simulink model "OLD_dec_fir_snb"  (R2012b)
settings: Solver=FixedStepDiscrete  SolverMode=SingleTasking  StartTime=0.0  StopTime=10000  FixedStep=1  RelTol=1e-3
libraries: xbsIndex_r4 x1157, casper_library_misc x5, xps_library x1
(part 1 of 9)
settings Model: Creator=paulp  LastModifiedBy=paulp
settings DataIOCC: LimitDataPoints=off
settings OptimizationCC: SimCompilerOptimization=On

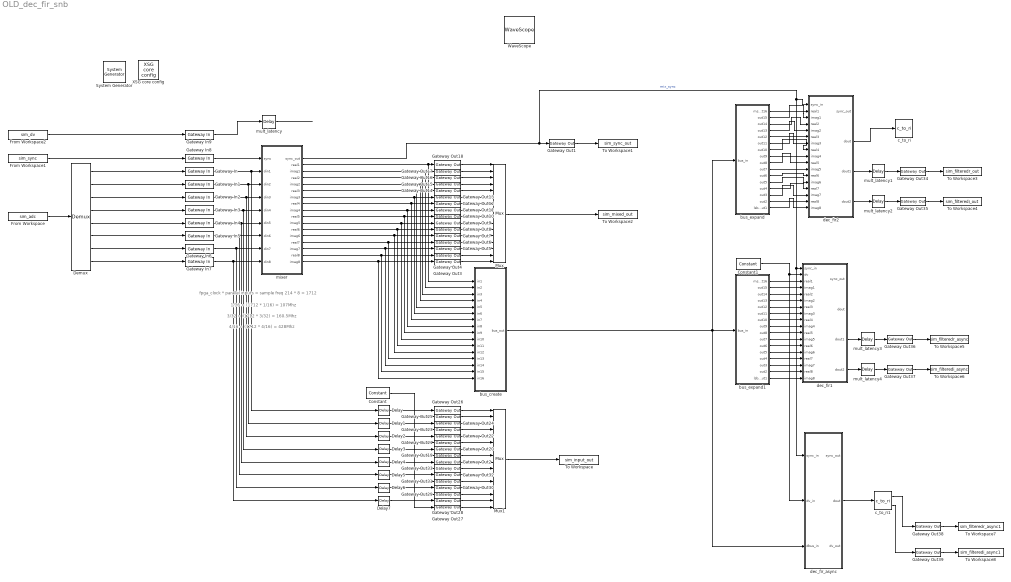
== system OLD_dec_fir_snb ==
  note: fpga_clock * parallel inputs = sample freq
      | 214 * 8 = 1712
  note: 1/16 = (1712 * 1/16) = 107Mhz
  note: 3/32 = (1712 * 3/32) = 160.5Mhz
  note: 4/16 = (1712 * 4/16) = 428Mhz
  " System Generator" : xbsIndex_r4/ System Generator  Tag=genX  xilinxfamily=virtex6  part=xc6vsx475t  speed=-1  package=ff1759  synthesis_tool=XST  clock_wrapper=Clock Enables  directory=./netlist  proj_type=Project Navigator  Synth_file=XST Defaults  Impl_file=ISE Defaults  testbench=off  simulink_period=1  sysclk_period=10  dcm_input_clock_period=10  incr_netlist=off  trim_vbits=Everywhere in SubSystem  dbl_ovrd=According to Block Masks  core_generation=According to Block Masks  run_coregen=off  deprecated_control=off  eval_field=0  block_type=sysgen
  Constant : xbsIndex_r4/Constant  const=0  gui_display_data_type=Fixed-point  arith_type=Signed (2's comp)  n_bits=10  bin_pt=9  preci_type=Single  exp_width=8  frac_width=24  explicit_period=on  period=1  equ=P=C  opselect=C  inp2=PCIN>>17  opr=+  inp1=P  carry=CIN  dbl_ovrd=off  block_type=constant
  Constant1 : xbsIndex_r4/Constant  const=1  gui_display_data_type=Boolean  arith_type=Boolean  n_bits=10  bin_pt=9  preci_type=Single  exp_width=8  frac_width=24  explicit_period=on  period=1  equ=P=C  opselect=C  inp2=PCIN>>17  opr=+  inp1=P  carry=CIN  dbl_ovrd=off  block_type=constant
  Delay{,1..7} (8 alike) : xbsIndex_r4/Delay  rst=off  infoeditControl=Selection of Reset will increase slice count due to use of real FFs and instead of SRLs  en=off  latency=1  dbl_ovrd=off  reg_retiming=off  block_type=delay
  Demux : Demux  Outputs=8
  From Workspace : FromWorkspace  VariableName=sim_adc  SampleTime=1  Interpolate=off  OutputAfterFinalValue=Setting to zero
  From Workspace1 : FromWorkspace  VariableName=sim_sync  SampleTime=1  Interpolate=off  OutputAfterFinalValue=Setting to zero
  From Workspace2 : FromWorkspace  VariableName=sim_dv  SampleTime=1  Interpolate=off  OutputAfterFinalValue=Setting to zero
  Gateway In{,1..7} (8 alike) : xbsIndex_r4/Gateway In  gui_display_data_type=Fixed-point  arith_type="Signed  (2's comp)"  n_bits=10  bin_pt=9  preci_type=Single  exp_width=8  frac_width=24  quantization="Round  (unbiased: +/- Inf)"  overflow=Saturate  period=1  dbl_ovrd=off  timing_constraint=None  locs_specified=off  LOCs={}  UseAsADC=off  ADCChannel='1'  inherit_from_input=off  hdl_port=on  block_type=gatewayin
  Gateway In8 : xbsIndex_r4/Gateway In  gui_display_data_type=Boolean  arith_type=Boolean  n_bits=10  bin_pt=9  preci_type=Single  exp_width=8  frac_width=24  quantization="Round  (unbiased: +/- Inf)"  overflow=Saturate  period=1  dbl_ovrd=off  timing_constraint=None  locs_specified=off  LOCs={}  UseAsADC=off  ADCChannel='1'  inherit_from_input=off  hdl_port=on  block_type=gatewayin
  Gateway In9 : xbsIndex_r4/Gateway In  gui_display_data_type=Boolean  arith_type=Boolean  n_bits=10  bin_pt=9  preci_type=Single  exp_width=8  frac_width=24  quantization="Round  (unbiased: +/- Inf)"  overflow=Saturate  period=1  dbl_ovrd=off  timing_constraint=None  locs_specified=off  LOCs={}  UseAsADC=off  ADCChannel='1'  inherit_from_input=off  hdl_port=on  block_type=gatewayin
  Gateway Out{1..39} (39 alike) : xbsIndex_r4/Gateway Out  inherit_from_input=off  hdl_port=off  timing_constraint=None  locs_specified=off  LOCs={}  UseAsDAC=off  DACChannel='1'  block_type=gatewayout
  Mux : Mux  Inputs=16
  Mux1 : Mux  Inputs=16
  To Workspace : ToWorkspace  VariableName=sim_input_out  SampleTime=1  SaveFormat=Structure With Time
  To Workspace1 : ToWorkspace  VariableName=sim_sync_out  SampleTime=1  SaveFormat=Structure With Time
  To Workspace2 : ToWorkspace  VariableName=sim_mixed_out  SampleTime=1  SaveFormat=Structure With Time
  To Workspace3 : ToWorkspace  VariableName=sim_filteredr_out  SampleTime=1  SaveFormat=Structure With Time
  To Workspace4 : ToWorkspace  VariableName=sim_filteredi_out  SampleTime=1  SaveFormat=Structure With Time
  To Workspace5 : ToWorkspace  VariableName=sim_filteredr_async  SampleTime=1  SaveFormat=Structure With Time
  To Workspace6 : ToWorkspace  VariableName=sim_filteredi_async  SampleTime=1  SaveFormat=Structure With Time
  To Workspace7 : ToWorkspace  VariableName=sim_filteredr_async1  SampleTime=1  SaveFormat=Structure With Time
  To Workspace8 : ToWorkspace  VariableName=sim_filteredi_async1  SampleTime=1  SaveFormat=Structure With Time
  WaveScope : xbsIndex_r4/WaveScope  block_type=wavescope
  XSG core config : xps_library/XSG core config  Tag=xps:xsg  hw_sys=ROACH2:sx475t  clk_src=sys_clk  ROACH_clk_src=sys_clk  ROACH2_clk_src=sys_clk  MKDIG_clk_src=sys_clk  clk_rate=214  sample_period=1  synthesis_tool=XST
  bus_create : Subsystem  AncestorBlock=casper_library_flow_control/bus_create  mask(bus_create){inputNum=16}
      mask prompts: inputNum "Number of inputs:"
      mask init:
      | bus_create_init(gcb,...
      |     'inputNum', inputNum);
  bus_expand : Subsystem  AncestorBlock=casper_library_flow_control/bus_expand  mask(bus_expand){mode=divisions of equal size, outputNum=16, outputWidth=20, outputBinaryPt=18, outputArithmeticType=1, show_format=off, outputToWorkspace=off, variablePrefix=out, outputToModelAsWell=on}
      mask prompts: outputNum "Number of outputs:"; outputWidth "Output width:"; outputBinaryPt "Output binary point position:"; outputArithmeticType "Output arithmetic type (ufix=0, fix=1, bool=2):"; show_format "Print format string?"; outputToWorkspace "Output to workspace?"; variablePrefix "Variable name prefix:"; outputToModelAsWell "Output to model as well?"
      mask help:
      | Expands a 'bus' made using a bus_create or Xilinx
      | concat block.
      | The input will be divided into the specified number
      | of outputs with the specified arithmetic types.
      | Divisions are made from most significant bit.
      mask init:
      | bus_expand_init(gcb,...
      |     'mode', mode, ...
      |     'outputNum', outputNum, ...
      |     'outputWidth', outputWidth, ...
      |     'outputBinaryPt', outputBinaryPt, ...
      |     'outputArithmeticType', outputArithmeticType, ...
      |     'show_format', show_format, ...
      |     'outputToWorkspace', outputToWorkspace, ...
      |     'variablePrefix', variablePrefix, ...
      |     'outputToModelAsWell', outputToModelAsWell);
      settings: AttributesFormatString=16 outputs
      mask TypeOptions mode: divisions of equal size | divisions of arbitrary size
      mask Callback mode: bus_expand_callback();
      mask Callback outputWidth: bus_expand_callback();
      mask Callback outputToWorkspace: bus_expand_callback();
  bus_expand1 : Subsystem  AncestorBlock=casper_library_flow_control/bus_expand  mask(bus_expand){mode=divisions of equal size, outputNum=16, outputWidth=20, outputBinaryPt=18, outputArithmeticType=1, show_format=off, outputToWorkspace=off, variablePrefix=out, outputToModelAsWell=on}
      mask prompts: outputNum "Number of outputs:"; outputWidth "Output width:"; outputBinaryPt "Output binary point position:"; outputArithmeticType "Output arithmetic type (ufix=0, fix=1, bool=2):"; show_format "Print format string?"; outputToWorkspace "Output to workspace?"; variablePrefix "Variable name prefix:"; outputToModelAsWell "Output to model as well?"
      mask help:
      | Expands a 'bus' made using a bus_create or Xilinx
      | concat block.
      | The input will be divided into the specified number
      | of outputs with the specified arithmetic types.
      | Divisions are made from most significant bit.
      mask init: same as OLD_dec_fir_snb/bus_expand
      settings: AttributesFormatString=16 outputs
      mask TypeOptions mode: divisions of equal size | divisions of arbitrary size
      mask Callback mode: bus_expand_callback();
      mask Callback outputWidth: bus_expand_callback();
      mask Callback outputToWorkspace: bus_expand_callback();
  c_to_ri : casper_library_misc/c_to_ri  n_bits=32  bin_pt=31
      settings: AttributesFormatString=32_31 r/i
  c_to_ri1 : casper_library_misc/c_to_ri  n_bits=20  bin_pt=19
      settings: AttributesFormatString=20_19 r/i
  dec_fir1 : Subsystem  Tag=casper:dec_fir  mask(dec_fir){n_inputs=8, coeff=|, n_bits=32, quantization=Round  (unbiased: +/- Inf), add_latency=1, mult_latency=2, conv_latency=2, coeff_bit_width=25, coeff_bin_pt=23, absorb_adders=off, adder_imp=Behavioral}
      mask coeff=|
      | [0.00192582027899352	0.00270863257211452	0.00460769136115305	0.00722478458223097	0.0106379289193187	0.0148769089466709	0.0199095287177559	0.0256326100943865	0.0318695836606276	0.0383758422175682	0.0448521125466397	0.0509650671776680	0.0563733906596148	0.0607566857782212	0.0638440864370335	0.0654393260500031	0.0654393260500031	0.0638440864370335	0.0607566857782212	0.0563733906596148	0.0509650671776680	0.0448521125466397	0.0383758422175682	0.0318695836606276	0.0256326100943865	0.0199095287177559	0.0148769089466709	0.0106379289193187	0.00722478458223097	0.00460769136115305	0.00270863257211452	0.00192582027899352
      | ]
      mask prompts: n_inputs "Number of Parallel Streams"; coeff "Coefficients"; n_bits "Bit Width Out"; quantization "Quantization Behavior"; add_latency "Add Latency"; mult_latency "Mult Latency"; conv_latency "Convert latency"; coeff_bit_width "Coefficient bit width"; coeff_bin_pt "Coefficient binary point"; absorb_adders "Absorb adders into DSP slices"; adder_imp "Adder implementation"
      mask help: FIR filter which can handle multiple time samples in parallel and decimates down to 1 time sample. If coefficients are symmetric, will automatically fold before multiplying.
      mask init:
      | % dec_fir_init(gcb, ...
      | %     'n_inputs', n_inputs, ...
      | %     'coeff', coeff, ...
      | %     'n_bits', n_bits, ...
      | %     'quantization', quantization, ...
      | %     'add_latency', add_latency, ...
      | %     'mult_latency', mult_latency, ...
      | %     'conv_latency', conv_latency, ...
      | %     'coeff_bit_width', coeff_bit_width, ...
      | %     'coeff_bin_pt', coeff_bin_pt, ...
      | %     'absorb_adders', absorb_adders, ...
      | %     'adder_imp', adder_imp);
      settings: AttributesFormatString=|
      | 32 taps
      | 32_31 r/i
      mask TypeOptions quantization: Truncate | Round  (unbiased: +/- Inf) | Round  (unbiased: Even Values)
      mask TypeOptions adder_imp: Behavioral | Fabric | DSP48
  dec_fir2 : Subsystem  Tag=casper:dec_fir  AncestorBlock=casper_library_downconverter/dec_fir  mask(dec_fir){n_inputs=8, coeff=|, n_bits=32, quantization=Round  (unbiased: +/- Inf), add_latency=1, mult_latency=2, conv_latency=2, coeff_bit_width=25, coeff_bin_pt=23, absorb_adders=off, adder_imp=Behavioral}
      mask coeff=|
      | [0.00192582027899352	0.00270863257211452	0.00460769136115305	0.00722478458223097	0.0106379289193187	0.0148769089466709	0.0199095287177559	0.0256326100943865	0.0318695836606276	0.0383758422175682	0.0448521125466397	0.0509650671776680	0.0563733906596148	0.0607566857782212	0.0638440864370335	0.0654393260500031	0.0654393260500031	0.0638440864370335	0.0607566857782212	0.0563733906596148	0.0509650671776680	0.0448521125466397	0.0383758422175682	0.0318695836606276	0.0256326100943865	0.0199095287177559	0.0148769089466709	0.0106379289193187	0.00722478458223097	0.00460769136115305	0.00270863257211452	0.00192582027899352
      | ]
      mask prompts: n_inputs "Number of Parallel Streams"; coeff "Coefficients"; n_bits "Bit Width Out"; quantization "Quantization Behavior"; add_latency "Add Latency"; mult_latency "Mult Latency"; conv_latency "Convert latency"; coeff_bit_width "Coefficient bit width"; coeff_bin_pt "Coefficient binary point"; absorb_adders "Absorb adders into DSP slices"; adder_imp "Adder implementation"
      mask help: FIR filter which can handle multiple time samples in parallel and decimates down to 1 time sample. If coefficients are symmetric, will automatically fold before multiplying.
      mask init:
      | dec_fir_init(gcb, ...
      |     'n_inputs', n_inputs, ...
      |     'coeff', coeff, ...
      |     'n_bits', n_bits, ...
      |     'quantization', quantization, ...
      |     'add_latency', add_latency, ...
      |     'mult_latency', mult_latency, ...
      |     'conv_latency', conv_latency, ...
      |     'coeff_bit_width', coeff_bit_width, ...
      |     'coeff_bin_pt', coeff_bin_pt, ...
      |     'absorb_adders', absorb_adders, ...
      |     'adder_imp', adder_imp);
      settings: AttributesFormatString=|
      | 32 taps
      | 32_31 r/i
      mask TypeOptions quantization: Truncate | Round  (unbiased: +/- Inf) | Round  (unbiased: Even Values)
      mask TypeOptions adder_imp: Behavioral | Fabric | DSP48
  dec_fir_async : Subsystem  Tag=casper:dec_fir_async  AncestorBlock=casper_library_downconverter/dec_fir_async  mask(dec_fir_async){n_inputs=8, coeff=|, output_width=20, output_bp=19, quantization=Round  (unbiased: +/- Inf), add_latency=1, mult_latency=2, conv_latency=2, coeff_bit_width=24, coeff_bin_pt=23, lshift=0, absorb_adders=off, adder_imp=Behavioral, async=on, bus_input=on, input_width=20, input_bp=18, input_type=Signed}
      mask coeff=|
      | [0.00192582027899352	0.00270863257211452	0.00460769136115305	0.00722478458223097	0.0106379289193187	0.0148769089466709	0.0199095287177559	0.0256326100943865	0.0318695836606276	0.0383758422175682	0.0448521125466397	0.0509650671776680	0.0563733906596148	0.0607566857782212	0.0638440864370335	0.0654393260500031	0.0654393260500031	0.0638440864370335	0.0607566857782212	0.0563733906596148	0.0509650671776680	0.0448521125466397	0.0383758422175682	0.0318695836606276	0.0256326100943865	0.0199095287177559	0.0148769089466709	0.0106379289193187	0.00722478458223097	0.00460769136115305	0.00270863257211452	0.00192582027899352
      | ]
      mask prompts: n_inputs "Number of Parallel Streams"; coeff "Coefficients"; output_width "Output bitwidth"; output_bp "Output binary point"; quantization "Quantization Behavior"; add_latency "Add Latency"; mult_latency "Mult Latency"; conv_latency "Convert latency"; coeff_bit_width "Coefficient bitwidth"; coeff_bin_pt "Coefficient binary point"; lshift "Post adder-tree shift"; absorb_adders "Absorb adders into DSP slices"; adder_imp "Adder implementation"; async "Asynchronous ops"; bus_input "Bus input"; input_width "Input bitwidth"; input_bp "Input binary point"; input_type "Input datatype"
      mask help: FIR filter which can handle multiple time samples in parallel and decimates down to 1 time sample. If coefficients are symmetric, will automatically fold before multiplying.
      mask init:
      | dec_fir_async_init(gcb);
      settings: AttributesFormatString=|
      | 32 taps
      | 20_19 r/i
      mask TypeOptions quantization: Truncate | Round  (unbiased: +/- Inf) | Round  (unbiased: Even Values)
      mask TypeOptions adder_imp: Behavioral | Fabric | DSP48
      mask Callback bus_input:
      | onoff = get_param(gcb, 'bus_input');
      | set_param_state(gcb, 'input_width', onoff)
      | set_param_state(gcb, 'input_bp', onoff)
      | set_param_state(gcb, 'input_type', onoff)
      mask TypeOptions input_type: Signed | Unsigned
  mixer : Subsystem  Tag=casper:mixer  AncestorBlock=casper_library_downconverter/mixer  mask(mixer){freq_div=16, freq=4, nstreams=8, n_bits=10, bram_latency=2, mult_latency=4}
      mask prompts: freq_div "Frequency Divisions (M)"; freq "Mixing Frequency (? / M*2pi)"; nstreams "Number of Parallel Streams"; n_bits "Bit Width"; bram_latency "BRAM Latency"; mult_latency "Mult Latency"
      mask help: Digitally mixes an input signal (which can be several samples in parallel) with an LO of the indicated frequency (which is some fraction of the native FPGA clock rate).
      mask init:
      | mixer_init(gcb, ...
      |     'freq_div', freq_div, ...
      |     'freq', freq, ...
      |     'nstreams', nstreams, ...
      |     'n_bits', n_bits, ...
      |     'bram_latency', bram_latency, ...
      |     'mult_latency', mult_latency);
      settings: AttributesFormatString=lo at -4/16
  mult_latency : xbsIndex_r4/Delay  rst=off  infoeditControl=Selection of Reset will increase slice count due to use of real FFs and instead of SRLs  en=off  latency=4  dbl_ovrd=off  reg_retiming=off  block_type=delay
  mult_latency{1..4} (4 alike) : xbsIndex_r4/Delay  rst=off  infoeditControl=Selection of Reset will increase slice count due to use of real FFs and instead of SRLs  en=off  latency=2  dbl_ovrd=off  reg_retiming=off  block_type=delay
  wires:
  From Workspace/1 -> Demux/1
  From Workspace1/1 -> Gateway In8/1
  Gateway In8/1 -> mixer/1(sync)
  Gateway In4/1 -> Delay4/1, mixer/6(din5)
  Gateway In3/1 -> Delay3/1, mixer/5(din4)
  Gateway In5/1 -> Delay5/1, mixer/7(din6)
  Gateway In6/1 -> Delay6/1, mixer/8(din7)
  Gateway In2/1 -> Delay2/1, mixer/4(din3)
  Gateway In7/1 -> Delay7/1, mixer/9(din8)
  Gateway In1/1 -> Delay1/1, mixer/3(din2)
  Gateway In/1 -> Delay/1, mixer/2(din1)
  Demux/1 -> Gateway In/1
  Demux/2 -> Gateway In1/1
  Demux/3 -> Gateway In2/1
  Demux/4 -> Gateway In3/1
  Demux/5 -> Gateway In4/1
  Demux/6 -> Gateway In5/1
  Demux/7 -> Gateway In6/1
  Demux/8 -> Gateway In7/1
  Gateway Out1/1 -> To Workspace1/1
  mixer/11(imag5) -> bus_create/10(in10), Gateway Out9/1
  mixer/12(real6) -> bus_create/11(in11), Gateway Out8/1
  mixer/13(imag6) -> bus_create/12(in12), Gateway Out7/1
  mixer/14(real7) -> bus_create/13(in13), Gateway Out6/1
  mixer/2(real1) -> bus_create/1(in1), Gateway Out18/1
  mixer/3(imag1) -> bus_create/2(in2), Gateway Out17/1
  mixer/4(real2) -> bus_create/3(in3), Gateway Out16/1
  mixer/5(imag2) -> bus_create/4(in4), Gateway Out15/1
  mixer/6(real3) -> bus_create/5(in5), Gateway Out14/1
  mixer/7(imag3) -> bus_create/6(in6), Gateway Out13/1
  mixer/8(real4) -> bus_create/7(in7), Gateway Out12/1
  mixer/9(imag4) -> bus_create/8(in8), Gateway Out11/1
  mixer/10(real5) -> bus_create/9(in9), Gateway Out10/1
  mixer/15(imag7) -> bus_create/14(in14), Gateway Out5/1
  mixer/16(real8) -> bus_create/15(in15), Gateway Out4/1
  mixer/17(imag8) -> bus_create/16(in16), Gateway Out3/1
  Gateway Out3/1 -> Mux/16
  Gateway Out4/1 -> Mux/15
  Gateway Out5/1 -> Mux/14
  Gateway Out6/1 -> Mux/13
  Gateway Out7/1 -> Mux/12
  Gateway Out8/1 -> Mux/11
  Gateway Out9/1 -> Mux/10
  Gateway Out10/1 -> Mux/9
  Gateway Out11/1 -> Mux/8
  Gateway Out12/1 -> Mux/7
  Gateway Out13/1 -> Mux/6
  Gateway Out14/1 -> Mux/5
  Gateway Out15/1 -> Mux/4
  Gateway Out16/1 -> Mux/3
  Gateway Out17/1 -> Mux/2
  Gateway Out18/1 -> Mux/1
  Gateway Out27/1 -> Mux1/16
  Gateway Out28/1 -> Mux1/15
  Gateway Out29/1 -> Mux1/14
  Gateway Out30/1 -> Mux1/13
  Gateway Out31/1 -> Mux1/12
  Gateway Out32/1 -> Mux1/11
  Gateway Out33/1 -> Mux1/10
  Gateway Out2/1 -> Mux1/9
  Gateway Out19/1 -> Mux1/8
  Gateway Out20/1 -> Mux1/7
  Gateway Out21/1 -> Mux1/6
  Gateway Out22/1 -> Mux1/5
  Gateway Out23/1 -> Mux1/4
  Gateway Out24/1 -> Mux1/3
  Gateway Out25/1 -> Mux1/2
  Gateway Out26/1 -> Mux1/1
  Constant/1 -> Gateway Out23/1, Gateway Out21/1, Gateway Out19/1, Gateway Out33/1, Gateway Out31/1, Gateway Out29/1, Gateway Out27/1, Gateway Out25/1
  Mux1/1 -> To Workspace/1
  Mux/1 -> To Workspace2/1
  Delay/1 -> Gateway Out26/1
  Delay1/1 -> Gateway Out24/1
  Delay2/1 -> Gateway Out22/1
  Delay3/1 -> Gateway Out20/1
  Delay4/1 -> Gateway Out2/1
  Delay5/1 -> Gateway Out32/1
  Delay6/1 -> Gateway Out30/1
  Delay7/1 -> Gateway Out28/1
  Gateway Out34/1 -> To Workspace3/1
  dec_fir2/2(dout) -> c_to_ri/1
  Gateway Out35/1 -> To Workspace4/1
  dec_fir2/3(dout1) -> mult_latency1/1
  dec_fir2/4(dout2) -> mult_latency2/1
  bus_expand/2(out15) -> dec_fir2/3(imag1)
  bus_expand/4(out13) -> dec_fir2/5(imag2)
  bus_expand/5(out12) -> dec_fir2/6(real3)
  bus_expand/16(lsb_out1) -> dec_fir2/17(imag8)
  bus_expand/10(out7) -> dec_fir2/11(imag5)
  bus_expand/12(out5) -> dec_fir2/13(imag6)
  bus_expand/3(out14) -> dec_fir2/4(real2)
  bus_expand/7(out10) -> dec_fir2/8(real4)
  bus_expand/8(out9) -> dec_fir2/9(imag4)
  bus_expand/14(out3) -> dec_fir2/15(imag7)
  bus_expand/6(out11) -> dec_fir2/7(imag3)
  bus_expand/11(out6) -> dec_fir2/12(real6)
  bus_expand/13(out4) -> dec_fir2/14(real7)
  bus_expand/15(out2) -> dec_fir2/16(real8)
  bus_expand/9(out8) -> dec_fir2/10(real5)
  bus_expand/1(msb_out16) -> dec_fir2/2(real1)
  mixer/1(sync_out) -> Gateway Out1/1, dec_fir_async/1(sync_in), dec_fir1/1(sync_in), dec_fir2/1(sync_in)  "mix_sync"
  bus_create/1(bus_out) -> dec_fir_async/3(dbus_in), bus_expand/1(bus_in), bus_expand1/1(bus_in)
  Gateway Out36/1 -> To Workspace5/1
  Gateway Out37/1 -> To Workspace6/1
  dec_fir1/3(dout1) -> mult_latency3/1
  dec_fir1/4(dout2) -> mult_latency4/1
  bus_expand1/2(out15) -> dec_fir1/4(imag1)
  bus_expand1/4(out13) -> dec_fir1/6(imag2)
  bus_expand1/5(out12) -> dec_fir1/7(real3)
  bus_expand1/16(lsb_out1) -> dec_fir1/18(imag8)
  bus_expand1/10(out7) -> dec_fir1/12(imag5)
  bus_expand1/12(out5) -> dec_fir1/14(imag6)
  bus_expand1/3(out14) -> dec_fir1/5(real2)
  bus_expand1/7(out10) -> dec_fir1/9(real4)
  bus_expand1/8(out9) -> dec_fir1/10(imag4)
  bus_expand1/14(out3) -> dec_fir1/16(imag7)
  bus_expand1/6(out11) -> dec_fir1/8(imag3)
  bus_expand1/11(out6) -> dec_fir1/13(real6)
  bus_expand1/13(out4) -> dec_fir1/15(real7)
  bus_expand1/15(out2) -> dec_fir1/17(real8)
  bus_expand1/9(out8) -> dec_fir1/11(real5)
  bus_expand1/1(msb_out16) -> dec_fir1/3(real1)
  Constant1/1 -> dec_fir_async/2(dv_in), dec_fir1/2(dv)
  From Workspace2/1 -> Gateway In9/1
  Gateway In9/1 -> mult_latency/1
  mult_latency/1 -> ?
  Gateway Out38/1 -> To Workspace7/1
  Gateway Out39/1 -> To Workspace8/1
  dec_fir_async/2(dout) -> c_to_ri1/1
  c_to_ri1/1 -> Gateway Out38/1
  c_to_ri1/2 -> Gateway Out39/1
  mult_latency1/1 -> Gateway Out34/1
  mult_latency2/1 -> Gateway Out35/1
  mult_latency3/1 -> Gateway Out36/1
  mult_latency4/1 -> Gateway Out37/1

== system OLD_dec_fir_snb/bus_create ==
  in1 : Inport
  in2 : Inport  Port=2
  in3 : Inport  Port=3
  in4 : Inport  Port=4
  in5 : Inport  Port=5
  in6 : Inport  Port=6
  in7 : Inport  Port=7
  in8 : Inport  Port=8
  in9 : Inport  Port=9
  in10 : Inport  Port=10
  in11 : Inport  Port=11
  in12 : Inport  Port=12
  in13 : Inport  Port=13
  in14 : Inport  Port=14
  in15 : Inport  Port=15
  in16 : Inport  Port=16
  concatenate : xbsIndex_r4/Concat  num_inputs=16  dbl_ovrd=off  block_type=concat
  reinterpret{1..16} (16 alike) : xbsIndex_r4/Reinterpret  force_arith_type=on  arith_type=Unsigned  force_bin_pt=on  bin_pt=0  block_type=reinterpret
      reinterpret1 settings: infoedit="Changes signal type without altering the binary representation.   You can changed the signal between signed and unsigned, and relocate the binary point.<br><br>Hardware notes: In hardware this block costs nothing.<br><br>Example:  Suppose the input is 6 bits wide, signed, with 2 fractional bits, and the output is forced to unsigned with 0 fractional bits.  Then an input of -2.0 (1110.00 in binary 2's complement) becomes an output of 56 (111000 in binary)."
      reinterpret2 settings: infoedit="Changes signal type without altering the binary representation.   You can changed the signal between signed and unsigned, and relocate the binary point.<br><br>Hardware notes: In hardware this block costs nothing.<br><br>Example:  Suppose the input is 6 bits wide, signed, with 2 fractional bits, and the output is forced to unsigned with 0 fractional bits.  Then an input of -2.0 (1110.00 in binary 2's complement) becomes an output of 56 (111000 in binary)."
  bus_out : Outport
  wires:
  concatenate/1 -> bus_out/1
  in1/1 -> reinterpret1/1
  reinterpret1/1 -> concatenate/1
  in2/1 -> reinterpret2/1
  reinterpret2/1 -> concatenate/2
  in3/1 -> reinterpret3/1
  reinterpret3/1 -> concatenate/3
  in4/1 -> reinterpret4/1
  reinterpret4/1 -> concatenate/4
  in5/1 -> reinterpret5/1
  reinterpret5/1 -> concatenate/5
  in6/1 -> reinterpret6/1
  reinterpret6/1 -> concatenate/6
  in7/1 -> reinterpret7/1
  reinterpret7/1 -> concatenate/7
  in8/1 -> reinterpret8/1
  reinterpret8/1 -> concatenate/8
  in9/1 -> reinterpret9/1
  reinterpret9/1 -> concatenate/9
  in10/1 -> reinterpret10/1
  reinterpret10/1 -> concatenate/10
  in11/1 -> reinterpret11/1
  reinterpret11/1 -> concatenate/11
  in12/1 -> reinterpret12/1
  reinterpret12/1 -> concatenate/12
  in13/1 -> reinterpret13/1
  reinterpret13/1 -> concatenate/13
  in14/1 -> reinterpret14/1
  reinterpret14/1 -> concatenate/14
  in15/1 -> reinterpret15/1
  reinterpret15/1 -> concatenate/15
  in16/1 -> reinterpret16/1
  reinterpret16/1 -> concatenate/16

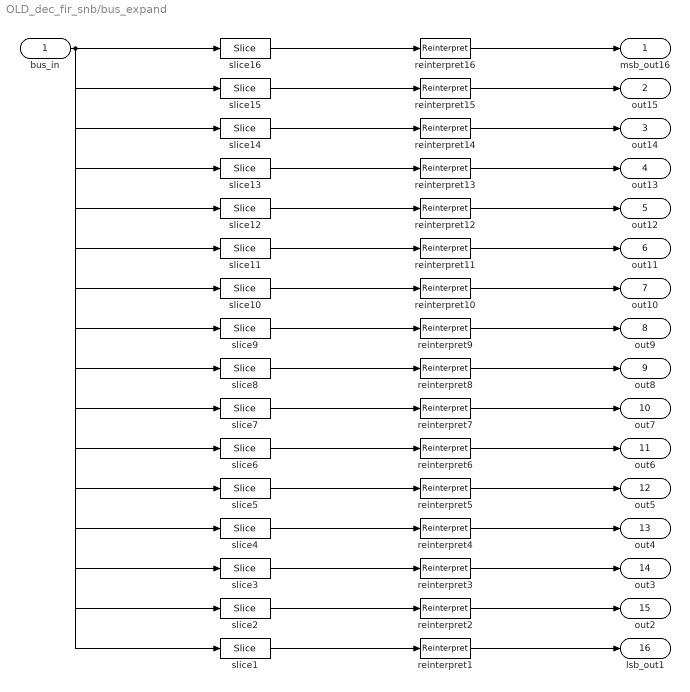
== system OLD_dec_fir_snb/bus_expand ==
  bus_in : Inport
  reinterpret{1..16} (16 alike) : xbsIndex_r4/Reinterpret  force_arith_type=on  arith_type="Signed  (2's comp)"  force_bin_pt=on  bin_pt=18  block_type=reinterpret
  slice1 : xbsIndex_r4/Slice  nbits=20  boolean_output=off  mode=Upper Bit Location + Width  bit1=-300  base1=MSB of Input  bit0=0  base0=LSB of Input  dbl_ovrd=off  block_type=slice
  slice10 : xbsIndex_r4/Slice  nbits=20  boolean_output=off  mode=Upper Bit Location + Width  bit1=-120  base1=MSB of Input  bit0=0  base0=LSB of Input  dbl_ovrd=off  block_type=slice
  slice11 : xbsIndex_r4/Slice  nbits=20  boolean_output=off  mode=Upper Bit Location + Width  bit1=-100  base1=MSB of Input  bit0=0  base0=LSB of Input  dbl_ovrd=off  block_type=slice
  slice12 : xbsIndex_r4/Slice  nbits=20  boolean_output=off  mode=Upper Bit Location + Width  bit1=-80  base1=MSB of Input  bit0=0  base0=LSB of Input  dbl_ovrd=off  block_type=slice
  slice13 : xbsIndex_r4/Slice  nbits=20  boolean_output=off  mode=Upper Bit Location + Width  bit1=-60  base1=MSB of Input  bit0=0  base0=LSB of Input  dbl_ovrd=off  block_type=slice
  slice14 : xbsIndex_r4/Slice  nbits=20  boolean_output=off  mode=Upper Bit Location + Width  bit1=-40  base1=MSB of Input  bit0=0  base0=LSB of Input  dbl_ovrd=off  block_type=slice
  slice15 : xbsIndex_r4/Slice  nbits=20  boolean_output=off  mode=Upper Bit Location + Width  bit1=-20  base1=MSB of Input  bit0=0  base0=LSB of Input  dbl_ovrd=off  block_type=slice
  slice16 : xbsIndex_r4/Slice  nbits=20  boolean_output=off  mode=Upper Bit Location + Width  bit1=0  base1=MSB of Input  bit0=0  base0=LSB of Input  dbl_ovrd=off  block_type=slice
  slice2 : xbsIndex_r4/Slice  nbits=20  boolean_output=off  mode=Upper Bit Location + Width  bit1=-280  base1=MSB of Input  bit0=0  base0=LSB of Input  dbl_ovrd=off  block_type=slice
  slice3 : xbsIndex_r4/Slice  nbits=20  boolean_output=off  mode=Upper Bit Location + Width  bit1=-260  base1=MSB of Input  bit0=0  base0=LSB of Input  dbl_ovrd=off  block_type=slice
  slice4 : xbsIndex_r4/Slice  nbits=20  boolean_output=off  mode=Upper Bit Location + Width  bit1=-240  base1=MSB of Input  bit0=0  base0=LSB of Input  dbl_ovrd=off  block_type=slice
  slice5 : xbsIndex_r4/Slice  nbits=20  boolean_output=off  mode=Upper Bit Location + Width  bit1=-220  base1=MSB of Input  bit0=0  base0=LSB of Input  dbl_ovrd=off  block_type=slice
  slice6 : xbsIndex_r4/Slice  nbits=20  boolean_output=off  mode=Upper Bit Location + Width  bit1=-200  base1=MSB of Input  bit0=0  base0=LSB of Input  dbl_ovrd=off  block_type=slice
  slice7 : xbsIndex_r4/Slice  nbits=20  boolean_output=off  mode=Upper Bit Location + Width  bit1=-180  base1=MSB of Input  bit0=0  base0=LSB of Input  dbl_ovrd=off  block_type=slice
  slice8 : xbsIndex_r4/Slice  nbits=20  boolean_output=off  mode=Upper Bit Location + Width  bit1=-160  base1=MSB of Input  bit0=0  base0=LSB of Input  dbl_ovrd=off  block_type=slice
  slice9 : xbsIndex_r4/Slice  nbits=20  boolean_output=off  mode=Upper Bit Location + Width  bit1=-140  base1=MSB of Input  bit0=0  base0=LSB of Input  dbl_ovrd=off  block_type=slice
  msb_out16 : Outport
  out15 : Outport  Port=2
  out14 : Outport  Port=3
  out13 : Outport  Port=4
  out12 : Outport  Port=5
  out11 : Outport  Port=6
  out10 : Outport  Port=7
  out9 : Outport  Port=8
  out8 : Outport  Port=9
  out7 : Outport  Port=10
  out6 : Outport  Port=11
  out5 : Outport  Port=12
  out4 : Outport  Port=13
  out3 : Outport  Port=14
  out2 : Outport  Port=15
  lsb_out1 : Outport  Port=16
  wires:
  bus_in/1 -> slice16/1, slice15/1, slice14/1, slice13/1, slice12/1, slice11/1, slice10/1, slice9/1, slice8/1, slice7/1, slice6/1, slice5/1, slice4/1, slice3/1, slice2/1, slice1/1
  slice16/1 -> reinterpret16/1
  reinterpret16/1 -> msb_out16/1
  slice15/1 -> reinterpret15/1
  reinterpret15/1 -> out15/1
  slice14/1 -> reinterpret14/1
  reinterpret14/1 -> out14/1
  slice13/1 -> reinterpret13/1
  reinterpret13/1 -> out13/1
  slice12/1 -> reinterpret12/1
  reinterpret12/1 -> out12/1
  slice11/1 -> reinterpret11/1
  reinterpret11/1 -> out11/1
  slice10/1 -> reinterpret10/1
  reinterpret10/1 -> out10/1
  slice9/1 -> reinterpret9/1
  reinterpret9/1 -> out9/1
  slice8/1 -> reinterpret8/1
  reinterpret8/1 -> out8/1
  slice7/1 -> reinterpret7/1
  reinterpret7/1 -> out7/1
  slice6/1 -> reinterpret6/1
  reinterpret6/1 -> out6/1
  slice5/1 -> reinterpret5/1
  reinterpret5/1 -> out5/1
  slice4/1 -> reinterpret4/1
  reinterpret4/1 -> out4/1
  slice3/1 -> reinterpret3/1
  reinterpret3/1 -> out3/1
  slice2/1 -> reinterpret2/1
  reinterpret2/1 -> out2/1
  slice1/1 -> reinterpret1/1
  reinterpret1/1 -> lsb_out1/1

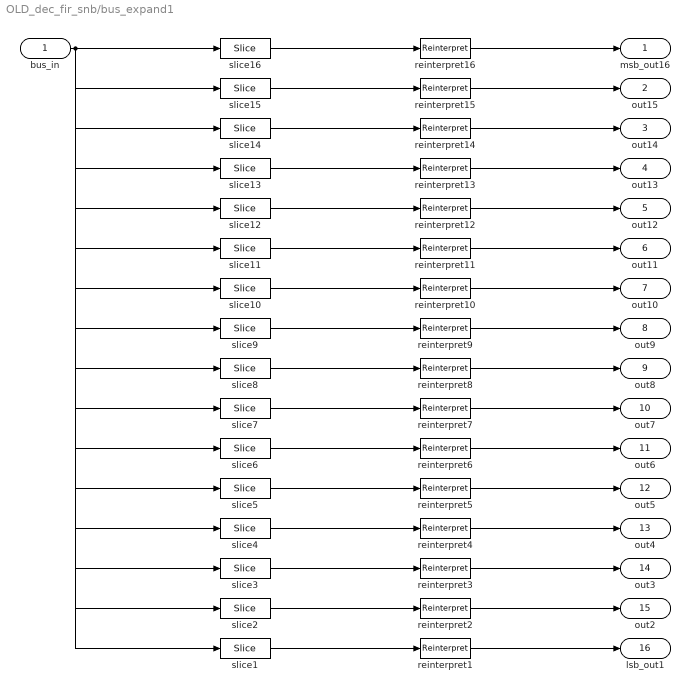
== system OLD_dec_fir_snb/bus_expand1 ==
  bus_in : Inport
  reinterpret{1..16} (16 alike) : xbsIndex_r4/Reinterpret  force_arith_type=on  arith_type="Signed  (2's comp)"  force_bin_pt=on  bin_pt=18  block_type=reinterpret
  slice1 : xbsIndex_r4/Slice  nbits=20  boolean_output=off  mode=Upper Bit Location + Width  bit1=-300  base1=MSB of Input  bit0=0  base0=LSB of Input  dbl_ovrd=off  block_type=slice
  slice10 : xbsIndex_r4/Slice  nbits=20  boolean_output=off  mode=Upper Bit Location + Width  bit1=-120  base1=MSB of Input  bit0=0  base0=LSB of Input  dbl_ovrd=off  block_type=slice
  slice11 : xbsIndex_r4/Slice  nbits=20  boolean_output=off  mode=Upper Bit Location + Width  bit1=-100  base1=MSB of Input  bit0=0  base0=LSB of Input  dbl_ovrd=off  block_type=slice
  slice12 : xbsIndex_r4/Slice  nbits=20  boolean_output=off  mode=Upper Bit Location + Width  bit1=-80  base1=MSB of Input  bit0=0  base0=LSB of Input  dbl_ovrd=off  block_type=slice
  slice13 : xbsIndex_r4/Slice  nbits=20  boolean_output=off  mode=Upper Bit Location + Width  bit1=-60  base1=MSB of Input  bit0=0  base0=LSB of Input  dbl_ovrd=off  block_type=slice
  slice14 : xbsIndex_r4/Slice  nbits=20  boolean_output=off  mode=Upper Bit Location + Width  bit1=-40  base1=MSB of Input  bit0=0  base0=LSB of Input  dbl_ovrd=off  block_type=slice
  slice15 : xbsIndex_r4/Slice  nbits=20  boolean_output=off  mode=Upper Bit Location + Width  bit1=-20  base1=MSB of Input  bit0=0  base0=LSB of Input  dbl_ovrd=off  block_type=slice
  slice16 : xbsIndex_r4/Slice  nbits=20  boolean_output=off  mode=Upper Bit Location + Width  bit1=0  base1=MSB of Input  bit0=0  base0=LSB of Input  dbl_ovrd=off  block_type=slice
  slice2 : xbsIndex_r4/Slice  nbits=20  boolean_output=off  mode=Upper Bit Location + Width  bit1=-280  base1=MSB of Input  bit0=0  base0=LSB of Input  dbl_ovrd=off  block_type=slice
  slice3 : xbsIndex_r4/Slice  nbits=20  boolean_output=off  mode=Upper Bit Location + Width  bit1=-260  base1=MSB of Input  bit0=0  base0=LSB of Input  dbl_ovrd=off  block_type=slice
  slice4 : xbsIndex_r4/Slice  nbits=20  boolean_output=off  mode=Upper Bit Location + Width  bit1=-240  base1=MSB of Input  bit0=0  base0=LSB of Input  dbl_ovrd=off  block_type=slice
  slice5 : xbsIndex_r4/Slice  nbits=20  boolean_output=off  mode=Upper Bit Location + Width  bit1=-220  base1=MSB of Input  bit0=0  base0=LSB of Input  dbl_ovrd=off  block_type=slice
  slice6 : xbsIndex_r4/Slice  nbits=20  boolean_output=off  mode=Upper Bit Location + Width  bit1=-200  base1=MSB of Input  bit0=0  base0=LSB of Input  dbl_ovrd=off  block_type=slice
  slice7 : xbsIndex_r4/Slice  nbits=20  boolean_output=off  mode=Upper Bit Location + Width  bit1=-180  base1=MSB of Input  bit0=0  base0=LSB of Input  dbl_ovrd=off  block_type=slice
  slice8 : xbsIndex_r4/Slice  nbits=20  boolean_output=off  mode=Upper Bit Location + Width  bit1=-160  base1=MSB of Input  bit0=0  base0=LSB of Input  dbl_ovrd=off  block_type=slice
  slice9 : xbsIndex_r4/Slice  nbits=20  boolean_output=off  mode=Upper Bit Location + Width  bit1=-140  base1=MSB of Input  bit0=0  base0=LSB of Input  dbl_ovrd=off  block_type=slice
  msb_out16 : Outport
  out15 : Outport  Port=2
  out14 : Outport  Port=3
  out13 : Outport  Port=4
  out12 : Outport  Port=5
  out11 : Outport  Port=6
  out10 : Outport  Port=7
  out9 : Outport  Port=8
  out8 : Outport  Port=9
  out7 : Outport  Port=10
  out6 : Outport  Port=11
  out5 : Outport  Port=12
  out4 : Outport  Port=13
  out3 : Outport  Port=14
  out2 : Outport  Port=15
  lsb_out1 : Outport  Port=16
  wires:
  reinterpret1/1 -> lsb_out1/1
  slice1/1 -> reinterpret1/1
  reinterpret2/1 -> out2/1
  slice2/1 -> reinterpret2/1
  reinterpret3/1 -> out3/1
  slice3/1 -> reinterpret3/1
  reinterpret4/1 -> out4/1
  slice4/1 -> reinterpret4/1
  reinterpret5/1 -> out5/1
  slice5/1 -> reinterpret5/1
  reinterpret6/1 -> out6/1
  slice6/1 -> reinterpret6/1
  reinterpret7/1 -> out7/1
  slice7/1 -> reinterpret7/1
  reinterpret8/1 -> out8/1
  slice8/1 -> reinterpret8/1
  reinterpret9/1 -> out9/1
  slice9/1 -> reinterpret9/1
  reinterpret10/1 -> out10/1
  slice10/1 -> reinterpret10/1
  reinterpret11/1 -> out11/1
  slice11/1 -> reinterpret11/1
  reinterpret12/1 -> out12/1
  slice12/1 -> reinterpret12/1
  reinterpret13/1 -> out13/1
  slice13/1 -> reinterpret13/1
  reinterpret14/1 -> out14/1
  slice14/1 -> reinterpret14/1
  reinterpret15/1 -> out15/1
  slice15/1 -> reinterpret15/1
  reinterpret16/1 -> msb_out16/1
  slice16/1 -> reinterpret16/1
  bus_in/1 -> slice1/1, slice2/1, slice3/1, slice4/1, slice5/1, slice6/1, slice7/1, slice8/1, slice9/1, slice10/1, slice11/1, slice12/1, slice13/1, slice14/1, slice15/1, slice16/1

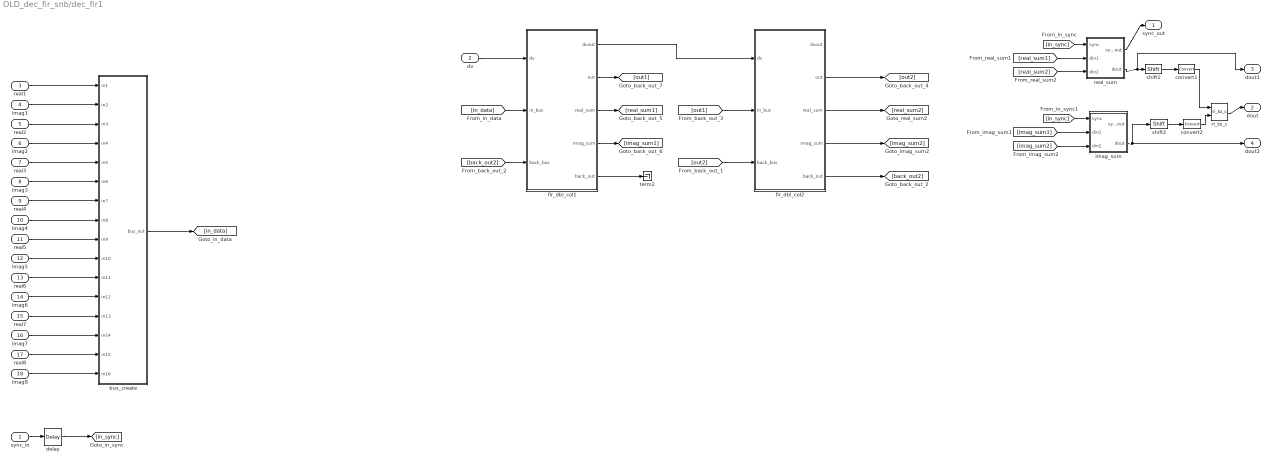
== system OLD_dec_fir_snb/dec_fir1 ==
  sync_in : Inport
  dv : Inport  Port=2
  real1 : Inport  Port=3
  imag1 : Inport  Port=4
  real2 : Inport  Port=5
  imag2 : Inport  Port=6
  real3 : Inport  Port=7
  imag3 : Inport  Port=8
  real4 : Inport  Port=9
  imag4 : Inport  Port=10
  real5 : Inport  Port=11
  imag5 : Inport  Port=12
  real6 : Inport  Port=13
  imag6 : Inport  Port=14
  real7 : Inport  Port=15
  imag7 : Inport  Port=16
  real8 : Inport  Port=17
  imag8 : Inport  Port=18
  bus_create : Subsystem  AncestorBlock=casper_library_flow_control/bus_create  mask(bus_create){inputNum=16}
      mask prompts: inputNum "Number of inputs:"
      mask init:
      | bus_create_init(gcb,...
      |     'inputNum', inputNum);
  convert1 : xbsIndex_r4/Convert  gui_display_data_type=Fixed-point  arith_type="Signed  (2's comp)"  n_bits=32  bin_pt=31  float_type=Single  exp_bits=8  fraction_bits=24  quantization="Round  (unbiased: +/- Inf)"  overflow=Wrap  en=off  latency=2  dbl_ovrd=off  pipeline=off  block_type=convert
  convert2 : xbsIndex_r4/Convert  gui_display_data_type=Fixed-point  arith_type="Signed  (2's comp)"  n_bits=32  bin_pt=31  float_type=Single  exp_bits=8  fraction_bits=24  quantization="Round  (unbiased: +/- Inf)"  overflow=Wrap  en=off  latency=2  dbl_ovrd=off  pipeline=off  block_type=convert
  delay : xbsIndex_r4/Delay  rst=off  infoeditControl=Selection of Reset will increase slice count due to use of real FFs and instead of SRLs  en=off  latency=8  dbl_ovrd=off  reg_retiming=off  block_type=delay
  fir_dbl_col1 : Subsystem  mask(fir_dbl_col){n_inputs=8, coeff=[0.025633     0.01991    0.014877    0.010638   0.0072248   0.0046077   0.0027086   0.0019258], add_latency=1, mult_latency=2, coeff_bit_width=25, coeff_bin_pt=23, first_stage_hdl=off, adder_imp=Behavioral}
      mask prompts: n_inputs "Inputs"; coeff "Coefficients"; add_latency "Add latency"; mult_latency "Mult Latency"; coeff_bit_width "Coefficient bit width"; coeff_bin_pt "Coefficient binary point"; first_stage_hdl "Implement first stage of adder trees on output as behavioural HDL"; adder_imp "Adder implementation"
      mask init:
      | % fir_dbl_col_init(gcb, ...
      | %     'n_inputs', n_inputs, ...
      | %     'coeff', coeff, ...
      | %     'mult_latency', mult_latency, ...
      | %     'add_latency', add_latency, ...
      | %     'coeff_bit_width', coeff_bit_width, ...
      | %     'coeff_bin_pt', coeff_bin_pt,  ...
      | %     'first_stage_hdl', first_stage_hdl, ...
      | %     'adder_imp', adder_imp);
      mask Help: eval('xlWeb(''http://casper.berkeley.edu/wiki/Fir_dbl_col'')')
      mask TypeOptions adder_imp: Behavioral | Fabric | DSP48
  fir_dbl_col2 : Subsystem  mask(fir_dbl_col){n_inputs=8, coeff=[0.065439    0.063844    0.060757    0.056373    0.050965    0.044852    0.038376     0.03187], add_latency=1, mult_latency=2, coeff_bit_width=25, coeff_bin_pt=23, first_stage_hdl=off, adder_imp=Behavioral}
      mask prompts: n_inputs "Inputs"; coeff "Coefficients"; add_latency "Add latency"; mult_latency "Mult Latency"; coeff_bit_width "Coefficient bit width"; coeff_bin_pt "Coefficient binary point"; first_stage_hdl "Implement first stage of adder trees on output as behavioural HDL"; adder_imp "Adder implementation"
      mask init: same as OLD_dec_fir_snb/dec_fir1/fir_dbl_col1
      mask Help: eval('xlWeb(''http://casper.berkeley.edu/wiki/Fir_dbl_col'')')
      mask TypeOptions adder_imp: Behavioral | Fabric | DSP48
  imag_sum : Subsystem  AncestorBlock=casper_library_misc/adder_tree  mask(adder_tree){n_inputs=2, latency=1, adder_imp=Behavioral, first_stage_hdl=off}
      mask prompts: n_inputs "Number of Inputs"; latency "Add Latency"; adder_imp "Adder implementation"; first_stage_hdl "Use behavioural HDL for first stage of adders"
      mask help:
      | Sums all inputs using a tree of adds and delays.
      |
      | Number of inputs: The number of inputs to the block to be summed
      | Add latency: The number of clock cycles to perform one addition (affects timing)..
      | Adder implementation: choice of fabric or DSP48E core, or behavioral HDL
      | Use behavioural HDL for first stage of adders: Causes the first stage of adders to be absorbed into DSP blocks if multipliers precede them (Virtex 5). Overrides Adder implementation
      mask init:
      | adder_tree_init(gcb, ...
      |     'n_inputs', n_inputs, ...
      |     'latency', latency, ...
      |     'adder_imp', adder_imp, ...
      |     'first_stage_hdl', first_stage_hdl);
      settings: AttributesFormatString=latency 1
      mask Help: eval('xlWeb(''http://casper.berkeley.edu/wiki/Adder_tree'')')
      mask TypeOptions adder_imp: Behavioral | Fabric | DSP48
  real_sum : Subsystem  AncestorBlock=casper_library_misc/adder_tree  mask(adder_tree){n_inputs=2, latency=1, adder_imp=Behavioral, first_stage_hdl=off}
      mask prompts: n_inputs "Number of Inputs"; latency "Add Latency"; adder_imp "Adder implementation"; first_stage_hdl "Use behavioural HDL for first stage of adders"
      mask help:
      | Sums all inputs using a tree of adds and delays.
      |
      | Number of inputs: The number of inputs to the block to be summed
      | Add latency: The number of clock cycles to perform one addition (affects timing)..
      | Adder implementation: choice of fabric or DSP48E core, or behavioral HDL
      | Use behavioural HDL for first stage of adders: Causes the first stage of adders to be absorbed into DSP blocks if multipliers precede them (Virtex 5). Overrides Adder implementation
      mask init:
      | adder_tree_init(gcb, ...
      |     'n_inputs', n_inputs, ...
      |     'latency', latency, ...
      |     'adder_imp', adder_imp, ...
      |     'first_stage_hdl', first_stage_hdl);
      settings: AttributesFormatString=latency 1
      mask Help: eval('xlWeb(''http://casper.berkeley.edu/wiki/Adder_tree'')')
      mask TypeOptions adder_imp: Behavioral | Fabric | DSP48
  ri_to_c : casper_library_misc/ri_to_c
  shift1 : xbsIndex_r4/Shift  shift_dir=Left  shift_bits=1  en=off  latency=0  precision=Full  arith_type="Signed  (2's comp)"  n_bits=16  bin_pt=14  quantization=Truncate  overflow=Wrap  dbl_ovrd=off  block_type=shift
  shift2 : xbsIndex_r4/Shift  shift_dir=Left  shift_bits=1  en=off  latency=0  precision=Full  arith_type="Signed  (2's comp)"  n_bits=16  bin_pt=14  quantization=Truncate  overflow=Wrap  dbl_ovrd=off  block_type=shift
  term2 : Terminator
  sync_out : Outport
  dout : Outport  Port=2
  dout1 : Outport  Port=3
  dout2 : Outport  Port=4
  wires:
  real_sum/1(sync_out) -> sync_out/1
  delay/1 -> [in_sync]
  sync_in/1 -> delay/1
  ri_to_c/1 -> dout/1
  convert2/1 -> ri_to_c/2
  convert1/1 -> ri_to_c/1
  shift2/1 -> convert2/1
  shift1/1 -> convert1/1
  imag_sum/2(dout) -> shift2/1, dout2/1
  real_sum/2(dout) -> shift1/1, dout1/1
  [in_sync] -> real_sum/1(sync)
  [in_sync] -> imag_sum/1(sync)
  fir_dbl_col1/5(back_out) -> term2/1
  real1/1 -> bus_create/1(in1)
  imag1/1 -> bus_create/2(in2)
  real2/1 -> bus_create/3(in3)
  imag2/1 -> bus_create/4(in4)
  real3/1 -> bus_create/5(in5)
  imag3/1 -> bus_create/6(in6)
  real4/1 -> bus_create/7(in7)
  imag4/1 -> bus_create/8(in8)
  real5/1 -> bus_create/9(in9)
  imag5/1 -> bus_create/10(in10)
  real6/1 -> bus_create/11(in11)
  imag6/1 -> bus_create/12(in12)
  real7/1 -> bus_create/13(in13)
  imag7/1 -> bus_create/14(in14)
  real8/1 -> bus_create/15(in15)
  imag8/1 -> bus_create/16(in16)
  fir_dbl_col2/5(back_out) -> [back_out2]
  [back_out2] -> fir_dbl_col1/3(back_bus)
  fir_dbl_col2/3(real_sum) -> [real_sum2]
  fir_dbl_col2/4(imag_sum) -> [imag_sum2]
  fir_dbl_col2/2(out) -> [out2]
  [out2] -> fir_dbl_col2/3(back_bus)
  fir_dbl_col1/3(real_sum) -> [real_sum1]
  fir_dbl_col1/4(imag_sum) -> [imag_sum1]
  fir_dbl_col1/2(out) -> [out1]
  [out1] -> fir_dbl_col2/2(in_bus)
  bus_create/1(bus_out) -> [in_data]
  [in_data] -> fir_dbl_col1/2(in_bus)
  dv/1 -> fir_dbl_col1/1(dv)
  [real_sum2] -> real_sum/3(din2)
  [imag_sum2] -> imag_sum/3(din2)
  [imag_sum1] -> imag_sum/2(din1)
  [real_sum1] -> real_sum/2(din1)
  fir_dbl_col1/1(dvout) -> fir_dbl_col2/1(dv)
